simulink model "SS_Kalman_Filter"  (R2019b)
settings: Solver=VariableStepAuto  StartTime=0.0  StopTime=60.0  FixedStep=0.00000001  RelTol=1e-3
undefined symbols (not defined in the file): __PRM__SERIALIZED__DATA__, pos, SubsystemReferenceBlock
settings Model: Creator=toons  LastModifiedBy=toons
settings DataIOCC: ExternalInput=[input1, input2]  ReturnWorkspaceOutputs=off
settings DebuggingCC: ArithmeticOperatorsInVariantConditions=warning
settings SFSimCC: CustomCodeUndefinedFunction=UseInterfaceOnly

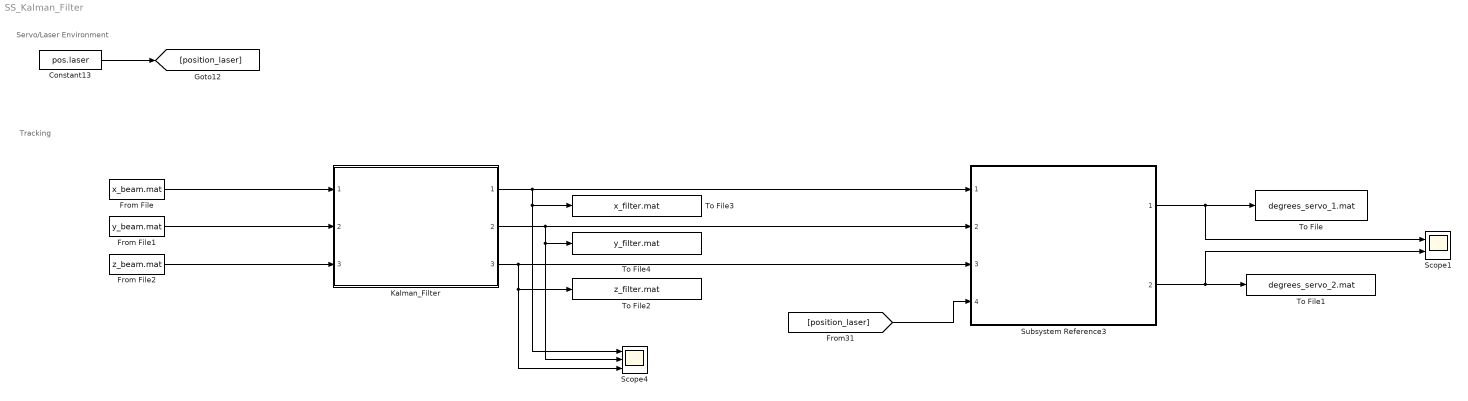
== system SS_Kalman_Filter ==
  note: Servo/Laser Environment
  note: Tracking
  Constant13 : Constant  Value=pos.laser  VectorParams1D=off
  From File : FromFile  FileName=x_beam.mat  SampleTime=0
  From File1 : FromFile  FileName=y_beam.mat  SampleTime=0
  From File2 : FromFile  FileName=z_beam.mat  SampleTime=0
  Kalman_Filter : Subsystem  BlockKeywords=__PRM__SERIALIZED__DATA__:SubsystemReferenceBlock  ReferencedSubsystem=Kalman_Filter
  Scope1 : Scope  NumInputPorts=2
  Scope4 : Scope  NumInputPorts=3
  Subsystem Reference3 : Subsystem  BlockKeywords=__PRM__SERIALIZED__DATA__:SubsystemReferenceBlock  ReferencedSubsystem=CartesianToServoDegrees
  To File : ToFile  Filename=degrees_servo_1.mat  SaveFormat=Timeseries
  To File1 : ToFile  Filename=degrees_servo_2.mat  SaveFormat=Timeseries
  To File2 : ToFile  Filename=z_filter.mat  SaveFormat=Timeseries
  To File3 : ToFile  Filename=x_filter.mat  SaveFormat=Timeseries
  To File4 : ToFile  Filename=y_filter.mat  SaveFormat=Timeseries
  wires:
  Kalman_Filter/1 -> Subsystem Reference3/1, To File3/1, Scope4/1
  Kalman_Filter/2 -> Subsystem Reference3/2, Scope4/2, To File4/1
  Kalman_Filter/3 -> Subsystem Reference3/3, Scope4/3, To File2/1
  Constant13/1 -> [position_laser]
  [position_laser] -> Subsystem Reference3/4
  From File/1 -> Kalman_Filter/1
  From File1/1 -> Kalman_Filter/2
  From File2/1 -> Kalman_Filter/3
  Subsystem Reference3/2 -> Scope1/2, To File1/1
  Subsystem Reference3/1 -> Scope1/1, To File/1
